simulink model "e7f"  (R2021a)
settings: Solver=VariableStepAuto  StartTime=0.0  StopTime=10.0  RelTol=1e-3
undefined symbols (not defined in the file or in its folder): strel
libraries: visionmorphops x4, visionconversions x3, visionsources x1
settings Model: Creator=pranshu  LastModifiedBy=pranshu

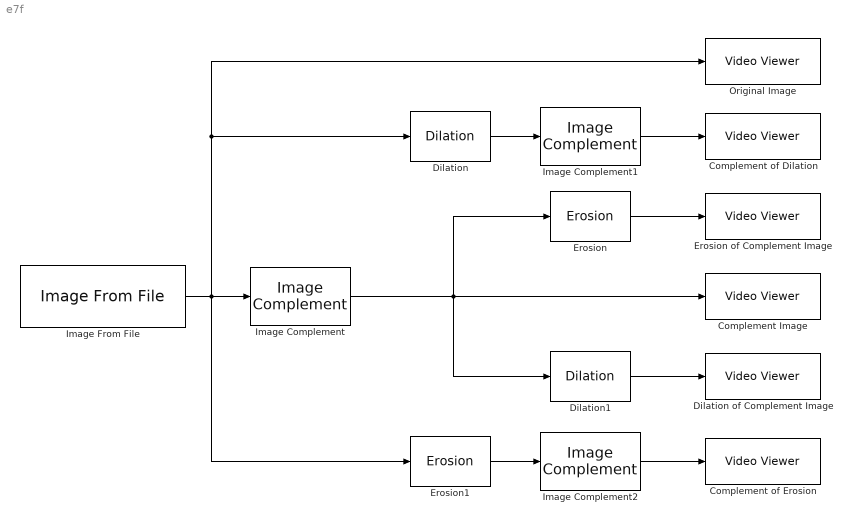
== system e7f ==
  Complement Image : VideoViewer  FigPos=[169.8 821.2 417.6 304]
  Complement of Dilation : VideoViewer  FigPos=[589 410 417.6 304]
  Complement of Erosion : VideoViewer  FigPos=[1008.2 410 417.6 304]
  Dilation : visionmorphops/Dilation  nhoodsrc=Specify via dialog  strel=[1 1; 1 1]
      settings: SourceProductBaseCode=VP
  Dilation of Complement Image : VideoViewer  FigPos=[1009 820.4 417.6 304]
  Dilation1 : visionmorphops/Dilation  nhoodsrc=Specify via dialog  strel=[1 1; 1 1]
      settings: SourceProductBaseCode=VP
  Erosion : visionmorphops/Erosion  nhoodsrc=Specify via dialog  strel=strel('square',4)
      settings: SourceProductBaseCode=VP
  Erosion of Complement Image : VideoViewer  FigPos=[589 821.2 417.6 304]
  Erosion1 : visionmorphops/Erosion  nhoodsrc=Specify via dialog  strel=strel('square',4)
      settings: SourceProductBaseCode=VP
  Image Complement : visionconversions/Image Complement
      settings: SourceProductBaseCode=VP
  Image Complement1 : visionconversions/Image Complement
      settings: SourceProductBaseCode=VP
  Image Complement2 : visionconversions/Image Complement
      settings: SourceProductBaseCode=VP
  Image From File : visionsources/Image From File  Tag=vipblks_nd  FileName=coins.png  Ts=inf  imagePorts=One multidimensional signal  OutPortLabels=R|G|B  ImageDataType=Inherit from input image  sdImageDataType=uint(8)  Signed=on  WordLength=16  FractionLengthMode=User-defined  FractionLength=15
  Original Image : VideoViewer  FigPos=[170.6 409.2 417.6 304]
  wires:
  Image From File/1 -> Erosion1/1, Original Image/1, Dilation/1, Image Complement/1
  Dilation/1 -> Image Complement1/1
  Image Complement1/1 -> Complement of Dilation/1
  Image Complement/1 -> Dilation1/1, Complement Image/1, Erosion/1
  Erosion/1 -> Erosion of Complement Image/1
  Erosion1/1 -> Image Complement2/1
  Image Complement2/1 -> Complement of Erosion/1
  Dilation1/1 -> Dilation of Complement Image/1
